simulink model "mod5counter"  (R2020a)
settings: Solver=ode45  StartTime=0.0  StopTime=50  RelTol=1e-3  EnableMultiTasking=on
settings Model: Creator=jrivitus  LastModifiedBy=I3
settings DataIOCC: LimitDataPoints=on  SaveFormat=Array  ReturnWorkspaceOutputs=off  SignalLoggingName=sigsOut
settings OptimizationCC: ExpressionDepthLimit=2147483647  InitFltsAndDblsToZero=on  EfficientMapNaN2IntZero=off  LifeSpan=inf
settings DebuggingCC: SaveWithParameterizedLinksMsg=none  UnderspecifiedInitializationDetection=Classic  MergeDetectMultiDrivingBlocksExec=none  SignalResolutionControl=TryResolveAllWithWarning  MultiTaskDSMMsg=warning  MultiTaskCondExecSysMsg=none  ParameterPrecisionLossMsg=none  FcnCallInpInsideContextMsg=warning  AllowSymbolicDim=off  StateNameClashWarn=warning  SFUnexpectedBacktrackingDiag=warning  SFNoUnconditionalDefaultTransitionDiag=warning  SFExecutionAtInitializationDiag=none  ArithmeticOperatorsInVariantConditions=warning
settings HardwareCC: ProdBitPerPointer=32  ProdBitPerSizeT=32  ProdBitPerPtrDiffT=32  ProdLargestAtomicFloat=None  ProdIntDivRoundTo=Undefined  ProdEndianess=Unspecified  ProdWordSize=32  ProdHWDeviceType=32-bit Generic  TargetUnknown=on
settings ModelReferenceCC: PropagateSignalLabelsOutOfModel=off
settings SFSimCC: SimUseLocalCustomCode=off  SimParseCustomCode=off
settings RTWCC: RTWUseLocalCustomCode=off
settings CodeAppCC: StateflowObjectComments=on
settings GRTTargetCC: TargetFcnLib=ansi_tfl_tmw.mat  TargetLangStandard=C89/C90 (ANSI)  CombineOutputUpdateFcns=off  GRTInterface=on
settings ConfigComp: CovMetricSettings=dw  CovHtmlReporting=on  CovSaveCumulativeToWorkspaceVar=on  CovSaveSingleToWorkspaceVar=on  CovExternalEMLEnable=off  CovSFcnEnable=off

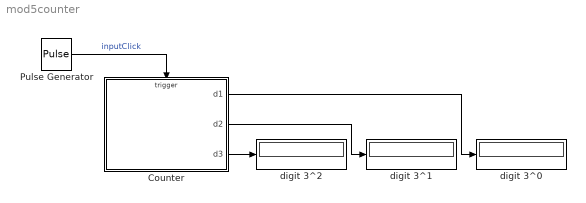
== system mod5counter ==
  Counter : Stateflow chart  TreatAsAtomicUnit=on
  Pulse Generator : DiscretePulseGenerator  PulseType=Time based  Period=10  PulseWidth=5
  digit 3^0 : Display
  digit 3^1 : Display
  digit 3^2 : Display
  wires:
  Counter/1(d1) -> digit 3^0/1
  Counter/2(d2) -> digit 3^1/1
  Counter/3(d3) -> digit 3^2/1
  Pulse Generator/1 -> Counter/Trigger  "inputClick"

== stateflow chart mod5counter/Counter ==
  settings: executeAtInitialization=1
  state digit1 [parallel]
    settings: executionOrder=1
    state one
      en: d1 = 1;
    state two
      en:
      d1=2;
    state three
      en:
      d1=3;
    state four
      en: d1 = 4;
    state zero
      en: d1 = 0;
    digit1.zero -> digit1.one : inputClick
    digit1.one -> digit1.two : inputClick
    digit1.two -> digit1.three : inputClick
    digit1.three -> digit1.four
    digit1.four -> digit1.zero : inputClick /{digit2.inc2;}
    (default) -> digit1.zero
  state digit2 [parallel]
    settings: executionOrder=2
    state one
      en: d2 = 1;
    state three
      en: d2 = 3;
    state two
      en: d2 = 2;
    state four
      en: d2 = 4;
    state zero
      en: d2 = 0;
    digit2.zero -> digit2.one : inc2
    digit2.one -> digit2.two : inc2
    digit2.two -> digit2.three : inc2
    digit2.three -> digit2.four : inc2
    (default) -> digit2.zero
    digit2.four -> digit2.zero : inc2 /{digit3.inc3;}
  state digit3 [parallel]
    settings: executionOrder=3
    state one
      en: d3 = 1;
    state two
      en: d2 = 2;
    state three
      en: d2 = 3;
    state four
      en: d3 = 4;
    state zero
      en: d3 = 0;
    digit3.zero -> digit3.one : inc3
    digit3.one -> digit3.two : inc3
    digit3.two -> digit3.three : inc3
    digit3.three -> digit3.four : inc3
    (default) -> digit3.zero
    digit3.four -> digit3.zero : inc3
  data: d1 output size=1; d2 output size=1; d3 output size=1
  events: inc2 local EITHER_EDGE_EVENT; inc3 local EITHER_EDGE_EVENT; inputClick input EITHER_EDGE_EVENT
